simulink model "myCellCharacterizationVerify"  (R2023a)
settings: Solver=daessc  StartTime=0.0  StopTime=2400  MaxStep=1  RelTol=1e-3  AbsTol=1e-3
InitFcn:
  | cellData=load('batt_BatteryCharacterizationResults_3s4p_2RC_20230929_1552.mat');fitData = cellData.battParameters{1,3};cellCapacity = cellData.battParameters{1,2};
undefined symbols (not defined in the file or in its folder): battery_builder_rtmsupport, gcbh
libraries: myPackFromBlock_lib x6, fl_lib x3, nesl_utility x3
CloseFcn:
  | clear fitData
settings Model: Creator=The MathWorks, Inc.  LastModifiedBy=paofu
settings SolverCC: AutoScaleAbsTol=off  AlgebraicLoopSolver=TrustRegion  MinimalZcImpactIntegration=on  MaxZcPerStep=1
settings OptimizationCC: ReuseModelBlockBuffer=off
settings DebuggingCC: ReadBeforeWriteMsg=DisableAll  WriteAfterWriteMsg=DisableAll  WriteAfterReadMsg=DisableAll  MultiTaskDSMMsg=none  UnconnectedInputMsg=warning  UnconnectedOutputMsg=warning  UnconnectedLineMsg=warning  SymbolicDimsDataTypeCodeGenerationDiagnostic=none
settings ModelReferenceCC: UpdateModelReferenceTargets=IfOutOfDate  EnableRefExpFcnMdlSchedulingChecks=on
settings SFSimCC: SFSimEcho=off  CustomCodeUndefinedFunction=UseInterfaceOnly
settings RTWCC: DLArmComputeVersion=19.05
settings SimscapeCC: SimscapeLogType=all  SimscapeLogSimulationStatistics=on  SimscapeLogName=simlog_CellCharacterizationVerify  SimscapeLogDataHistory=10000

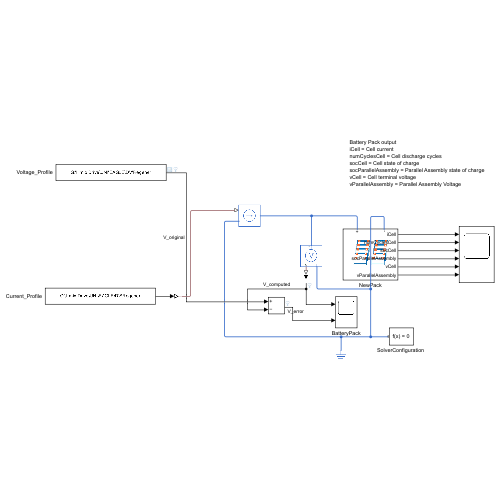
[thumbnail: Simulink's stored preview of the top-level diagram]
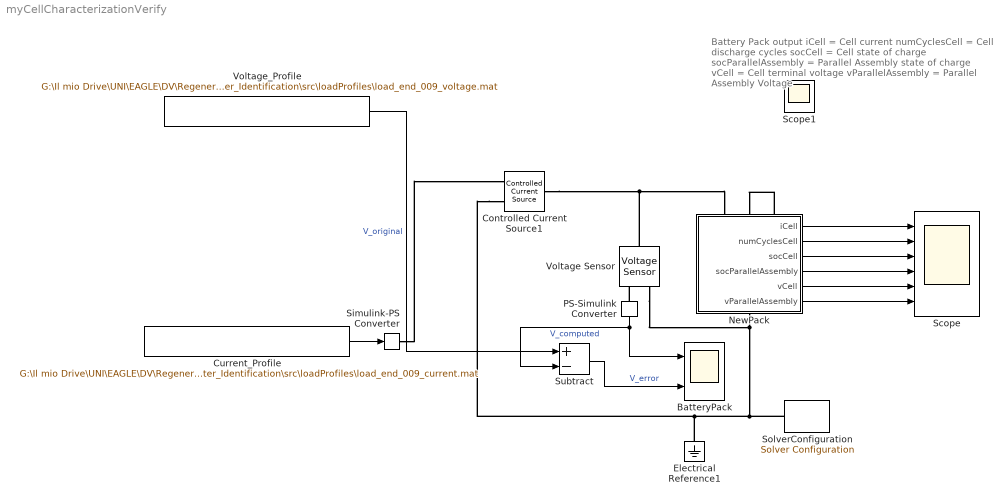
== system myCellCharacterizationVerify ==
  note: Battery Pack output
      | iCell = Cell current
      | numCyclesCell = Cell discharge cycles
      | socCell = Cell state of charge
      | socParallelAssembly = Parallel Assembly state of charge
      | vCell = Cell terminal voltage
      | vParallelAssembly = Parallel Assembly Voltage
  BatteryPack : Scope  NumInputPorts=2
  Controlled Current Source1 : fl_lib/Electrical/Electrical Sources/Controlled Current Source
  Current_Profile : FromFile  FileName=G:\Il mio Drive\UNI\EAGLE\DV\Regenerative-Braking-Development\MATLAB\Parameter_Identification\src\loadProfiles\load_end_009_current.mat  SampleTime=0
  Electrical Reference1 : fl_lib/Electrical/Electrical Elements/Electrical Reference
  NewPack : Subsystem  LoadFcn=battery_builder_rtmsupport('loadfcn',gcbh);
      settings: CopyFcn=battery_builder_rtmsupport('copyfcn',gcbh);  PreCopyFcn=battery_builder_rtmsupport('precopyfcn',gcbh);  PreDeleteFcn=battery_builder_rtmsupport('predeletefcn',gcbh);  PortSchema="{\"entries\":[{\"content\":{\"sides\":[{\"content\":{\"connectorIds\":[\"LConn1\",\"LConn2\"]},\"type\":\"ConnectorPlacement.EquallySpacedRectSide\",\"uuid\":\"66086b7d-23cd-42c5-ba93-ecc496197d21\"},{\"content\":{\"side\":\"RIGHT\"},\"type\":\"ConnectorPlacement.EquallySpacedRectSide\",\"uuid\":\"5adac210-02d4-41ca-984c-4f933a9ee7b3\"},{\"content\":{\"side\":\"TOP\"},\"type\":\"ConnectorPlacement.EquallySpacedRectSide\",\"uuid\":\"5928a5bb-4e09-460c-90ed-8eef0369e6eb\"},{\"content\":{\"connectorIds\":[\"Out1\",\"Out2\",\"Out3\",\"Out4\",\"Out5\",\"Out6\"],\"side\":\"BOTTOM\"},\"type\":\"ConnectorPlacement.EquallySpacedRectSide\",\"uuid\":\"b51498ad-47de-436d-ad23-9534549e135d\"}]},\"type\":\"ConnectorPlacement.EquallySpacedConnector\",\"uuid\":\"4448a3cb-869d-481a-9f4f-41a9fd16508a\"}],\"packageUris\":[\"http://schema.mathworks.com/mf0/Connector/R2020b\"],\"version\":\"1.0\"}"
      mask Display: image('$imagefile')
  PS-Simulink Converter : nesl_utility/PS-Simulink Converter  PhysicalDomain=network_engine_domain  SubClassName=ps_output  LeftPortType=input  RightPortType=output  PseudoPeriodic=off  Frequencies=[]  VectorFormat=inherit  Unit=inherit  AffineConversion=off
  Scope : Scope  NumInputPorts=6
  Simulink-PS Converter : nesl_utility/Simulink-PS Converter  PhysicalDomain=network_engine_domain  SubClassName=ps_input  LeftPortType=input  RightPortType=output  PseudoPeriodic=off  Frequencies=[]  NoiseDistribution=none  NoiseParameters=[]  Unit=1  AffineConversion=off  FilteringAndDerivatives=provide  SimscapeFilterOrder=1  InputFilterTimeConstant=0.001  UdotUserProvided=0
  "SolverConfiguration " : nesl_utility/Solver Configuration  PhysicalDomain=network_engine_domain  SubClassName=solver  LeftPortType=input  RightPortType=generic  Tones=[]  Harmonics=[]  SimulateNoise=off  Profile=off  UseLocalSampling=off  EnableSwitchedLinearOptims=on  FrequencyDomain=off  UseCCode=off  RelTol=0.001  AbsTol=1e-06  MinStep=1e-09  ToWorkspace=off  RevertToSquareIcSolve=off  NumHomotopyIterations=100  PhasorMode=off  PhasorModeNumHarmonics=1  ConsistencySolver=NEWTON_XTOL_AFTER_FTOL  IndexReductionMethod=DerivativeReplacement  DoDC=off  ResidualTolerance=1e-09  ConsistencyTolSource=GLOBAL  ConsistencyAbsTol=0.001  ConsistencyRelTol=0.001  ConsistencyTolFactor=0.001  UseLocalSolver=off  LocalSolverChoice=NE_BACKWARD_EULER_ADVANCER  ResolveIndetEquations=on  FunctionEvalNumThread=1  LocalSolverSampleTime=0.001  DoFixedCost=off  MaxNonlinIter=3  MaxModeIter=2  ComputeImpulses=off  ImpulseIterations=2  LinearAlgebra=auto  LinearAlgebraNumThread=0  EquationFormulation=NE_TIME_EF  DelaysMemoryBudget=1024  AutomaticFiltering=on  FilteringTimeConstant=0.001  PartitionStorageMethod=AS_NEEDED  PartitionMemoryBudget=1024  PartitionMethod=ROBUST
  Subtract : Sum  Inputs=+-
  Voltage Sensor : fl_lib/Electrical/Electrical Sensors/Voltage Sensor
  Voltage_Profile : FromFile  FileName=G:\Il mio Drive\UNI\EAGLE\DV\Regenerative-Braking-Development\MATLAB\Parameter_Identification\src\loadProfiles\load_end_009_voltage.mat  SampleTime=0
  Scope1 : Scope
  wires:
  NewPack/1(iCell) -> Scope/1
  NewPack/2(numCyclesCell) -> Scope/2
  NewPack/3(socCell) -> Scope/3
  NewPack/4(socParallelAssembly) -> Scope/4
  NewPack/5(vCell) -> Scope/5
  NewPack/6(vParallelAssembly) -> Scope/6
  Current_Profile/1 -> Simulink-PS Converter/1
  PS-Simulink Converter/1 -> BatteryPack/1, Subtract/2  "V_computed"
  Subtract/1 -> BatteryPack/2  "V_error"
  Voltage_Profile/1 -> Subtract/1  "V_original"
  connections:
  Controlled Current Source1/RConn2 -- Electrical Reference1/LConn1 -- Voltage Sensor/RConn2 -- NewPack/LConn2 -- "SolverConfiguration "/RConn1
  Simulink-PS Converter/RConn1 -- Controlled Current Source1/RConn1
  Voltage Sensor/LConn1 -- Controlled Current Source1/LConn1 -- NewPack/LConn1
  PS-Simulink Converter/LConn1 -- Voltage Sensor/RConn1

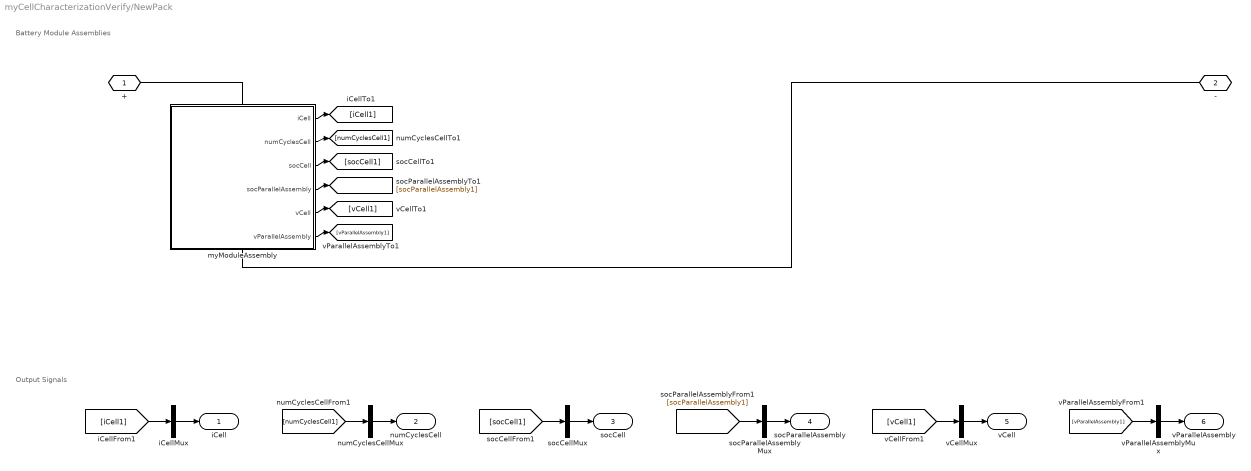
== system myCellCharacterizationVerify/NewPack ==
  note: Battery Module Assemblies
  note: Output Signals
  iCellMux : Mux  Inputs=1
  myModuleAssembly : Subsystem  LoadFcn=battery_builder_rtmsupport('loadfcn',gcbh);
      settings: CopyFcn=battery_builder_rtmsupport('copyfcn',gcbh);  PreCopyFcn=battery_builder_rtmsupport('precopyfcn',gcbh);  PreDeleteFcn=battery_builder_rtmsupport('predeletefcn',gcbh);  PortSchema="{\"entries\":[{\"content\":{\"sides\":[{\"content\":{\"connectorIds\":[\"LConn1\"]},\"type\":\"ConnectorPlacement.EquallySpacedRectSide\",\"uuid\":\"66086b7d-23cd-42c5-ba93-ecc496197d21\"},{\"content\":{\"connectorIds\":[\"RConn1\"],\"side\":\"RIGHT\"},\"type\":\"ConnectorPlacement.EquallySpacedRectSide\",\"uuid\":\"5adac210-02d4-41ca-984c-4f933a9ee7b3\"},{\"content\":{\"side\":\"TOP\"},\"type\":\"ConnectorPlacement.EquallySpacedRectSide\",\"uuid\":\"5928a5bb-4e09-460c-90ed-8eef0369e6eb\"},{\"content\":{\"connectorIds\":[\"Out1\",\"Out2\",\"Out3\",\"Out4\",\"Out5\",\"Out6\"],\"side\":\"BOTTOM\"},\"type\":\"ConnectorPlacement.EquallySpacedRectSide\",\"uuid\":\"b19a6cd0-397b-400c-bc99-badf0012d139\"}]},\"type\":\"ConnectorPlacement.EquallySpacedConnector\",\"uuid\":\"4448a3cb-869d-481a-9f4f-41a9fd16508a\"}],\"packageUris\":[\"http://schema.mathworks.com/mf0/Connector/R2020b\"],\"version\":\"1.0\"}"
      mask Display: image('$imagefile')
  numCyclesCellMux : Mux  Inputs=1
  socCellMux : Mux  Inputs=1
  socParallelAssemblyMux : Mux  Inputs=1
  vCellMux : Mux  Inputs=1
  vParallelAssemblyMux : Mux  Inputs=1
  + : PMIOPort  Side=Left
  - : PMIOPort  Port=2  Side=Left
  iCell : Outport
  numCyclesCell : Outport  Port=2
  socCell : Outport  Port=3
  socParallelAssembly : Outport  Port=4
  vCell : Outport  Port=5
  vParallelAssembly : Outport  Port=6
  wires:
  myModuleAssembly/1(iCell) -> [iCell1]
  iCellMux/1 -> iCell/1
  [iCell1] -> iCellMux/1
  myModuleAssembly/2(numCyclesCell) -> [numCyclesCell1]
  numCyclesCellMux/1 -> numCyclesCell/1
  [numCyclesCell1] -> numCyclesCellMux/1
  myModuleAssembly/3(socCell) -> [socCell1]
  socCellMux/1 -> socCell/1
  [socCell1] -> socCellMux/1
  myModuleAssembly/4(socParallelAssembly) -> [socParallelAssembly1]
  socParallelAssemblyMux/1 -> socParallelAssembly/1
  [socParallelAssembly1] -> socParallelAssemblyMux/1
  myModuleAssembly/5(vCell) -> [vCell1]
  vCellMux/1 -> vCell/1
  [vCell1] -> vCellMux/1
  myModuleAssembly/6(vParallelAssembly) -> [vParallelAssembly1]
  vParallelAssemblyMux/1 -> vParallelAssembly/1
  [vParallelAssembly1] -> vParallelAssemblyMux/1
  connections:
  myModuleAssembly/LConn1 -- +/RConn1
  myModuleAssembly/RConn1 -- -/RConn1

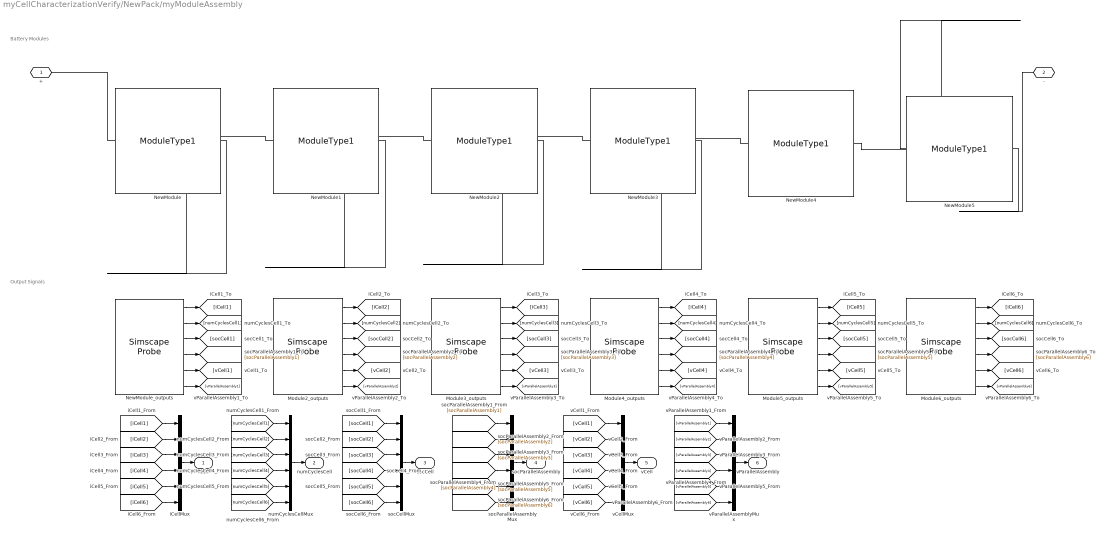
== system myCellCharacterizationVerify/NewPack/myModuleAssembly ==
  note: Output Signals
  note: Battery Modules
  Module2_outputs : SimscapeProbe  BoundBlock=328  Variables={iCell, numCyclesCell, socCell, socParallelAssembly, vCell, vParallelAssembly}
  Module3_outputs : SimscapeProbe  BoundBlock=329  Variables={iCell, numCyclesCell, socCell, socParallelAssembly, vCell, vParallelAssembly}
  Module4_outputs : SimscapeProbe  BoundBlock=330  Variables={iCell, numCyclesCell, socCell, socParallelAssembly, vCell, vParallelAssembly}
  Module5_outputs : SimscapeProbe  BoundBlock=331  Variables={iCell, numCyclesCell, socCell, socParallelAssembly, vCell, vParallelAssembly}
  Module6_outputs : SimscapeProbe  BoundBlock=332  Variables={iCell, numCyclesCell, socCell, socParallelAssembly, vCell, vParallelAssembly}
  NewModule{,1..5} (6 alike) : myPackFromBlock_lib/Modules/ModuleType1  SOC_vecCell=fitData.SOC  V0_vecCell=fitData.V0 V  V_rangeCell=[0, inf] V  R0_vecCell=(fitData.R0_charge + fitData.R0_discharge)/2 Ohm  AHCell=cellCapacity A*hr  extrapolation_optionCell=simscape.enum.extrapolation.nearest  R1_vecCell=fitData.R1 Ohm  tau1_vecCell=fitData.Tau1 s  R2_vecCell=fitData.R2 Ohm  tau2_vecCell=fitData.Tau2 s  P=1  S=6  iCell_specify=off  iCell_priority=None  iCell=0 A  iCell_nominal_specify=off  iCell_nominal_unit=A  iCell_nominal_value=1  vCell_specify=off  vCell_priority=None  vCell=0 V  vCell_nominal_specify=off  vCell_nominal_unit=V  vCell_nominal_value=1  socCell_specify=off  socCell_priority=High  socCell=1  socCell_nominal_specify=off  socCell_nominal_unit=1  socCell_nominal_value=1  numCyclesCell_specify=off  numCyclesCell_priority=High  numCyclesCell=0  numCyclesCell_nominal_specify=off  numCyclesCell_nominal_unit=1  numCyclesCell_nominal_value=1  vParallelAssembly_specify=off  vParallelAssembly_priority=None  vParallelAssembly=repmat(0, 6, 1) V  vParallelAssembly_nominal_specify=off  vParallelAssembly_nominal_unit=V  vParallelAssembly_nominal_value=1  socParallelAssembly_specify=off  socParallelAssembly_priority=None  socParallelAssembly=repmat(1, 6, 1)  socParallelAssembly_nominal_specify=off  socParallelAssembly_nominal_unit=1  socParallelAssembly_nominal_value=1
      settings: InternalSimscapePortConfiguration="{\"Bottom\":[{\"id\":\"n\",\"label\":\"-\",\"type\":\"foundation.electrical.electrical\"}],\"Left\":[],\"Right\":[],\"Top\":[{\"id\":\"p\",\"label\":\"+\",\"type\":\"foundation.electrical.electrical\"}]}"
  NewModule_outputs : SimscapeProbe  BoundBlock=213  Variables={iCell, numCyclesCell, socCell, socParallelAssembly, vCell, vParallelAssembly}
  iCellMux : Mux  Inputs=6
  numCyclesCellMux : Mux  Inputs=6
  socCellMux : Mux  Inputs=6
  socParallelAssemblyMux : Mux  Inputs=6
  vCellMux : Mux  Inputs=6
  vParallelAssemblyMux : Mux  Inputs=6
  + : PMIOPort  Side=Left
  - : PMIOPort  Port=2  Side=Right
  iCell : Outport
  numCyclesCell : Outport  Port=2
  socCell : Outport  Port=3
  socParallelAssembly : Outport  Port=4
  vCell : Outport  Port=5
  vParallelAssembly : Outport  Port=6
  wires:
  [vParallelAssembly6] -> vParallelAssemblyMux/6
  Module6_outputs/6 -> [vParallelAssembly6]
  [vCell6] -> vCellMux/6
  Module6_outputs/5 -> [vCell6]
  [socParallelAssembly6] -> socParallelAssemblyMux/6
  Module6_outputs/4 -> [socParallelAssembly6]
  [socCell6] -> socCellMux/6
  Module6_outputs/3 -> [socCell6]
  [numCyclesCell6] -> numCyclesCellMux/6
  Module6_outputs/2 -> [numCyclesCell6]
  [iCell6] -> iCellMux/6
  Module6_outputs/1 -> [iCell6]
  [vParallelAssembly5] -> vParallelAssemblyMux/5
  [vCell5] -> vCellMux/5
  [socParallelAssembly5] -> socParallelAssemblyMux/5
  [socCell5] -> socCellMux/5
  [numCyclesCell5] -> numCyclesCellMux/5
  [iCell5] -> iCellMux/5
  [vParallelAssembly4] -> vParallelAssemblyMux/4
  [vCell4] -> vCellMux/4
  [socParallelAssembly4] -> socParallelAssemblyMux/4
  [socCell4] -> socCellMux/4
  [numCyclesCell4] -> numCyclesCellMux/4
  [iCell4] -> iCellMux/4
  [vParallelAssembly3] -> vParallelAssemblyMux/3
  [vCell3] -> vCellMux/3
  [socParallelAssembly3] -> socParallelAssemblyMux/3
  [socCell3] -> socCellMux/3
  [numCyclesCell3] -> numCyclesCellMux/3
  [iCell3] -> iCellMux/3
  [vParallelAssembly2] -> vParallelAssemblyMux/2
  [vCell2] -> vCellMux/2
  [socParallelAssembly2] -> socParallelAssemblyMux/2
  [socCell2] -> socCellMux/2
  [numCyclesCell2] -> numCyclesCellMux/2
  [iCell2] -> iCellMux/2
  [vParallelAssembly1] -> vParallelAssemblyMux/1
  vParallelAssemblyMux/1 -> vParallelAssembly/1
  NewModule_outputs/6 -> [vParallelAssembly1]
  [vCell1] -> vCellMux/1
  vCellMux/1 -> vCell/1
  NewModule_outputs/5 -> [vCell1]
  [socParallelAssembly1] -> socParallelAssemblyMux/1
  socParallelAssemblyMux/1 -> socParallelAssembly/1
  NewModule_outputs/4 -> [socParallelAssembly1]
  [socCell1] -> socCellMux/1
  socCellMux/1 -> socCell/1
  NewModule_outputs/3 -> [socCell1]
  [numCyclesCell1] -> numCyclesCellMux/1
  numCyclesCellMux/1 -> numCyclesCell/1
  NewModule_outputs/2 -> [numCyclesCell1]
  [iCell1] -> iCellMux/1
  iCellMux/1 -> iCell/1
  NewModule_outputs/1 -> [iCell1]
  Module2_outputs/1 -> [iCell2]
  Module2_outputs/2 -> [numCyclesCell2]
  Module2_outputs/3 -> [socCell2]
  Module2_outputs/4 -> [socParallelAssembly2]
  Module2_outputs/5 -> [vCell2]
  Module2_outputs/6 -> [vParallelAssembly2]
  Module3_outputs/1 -> [iCell3]
  Module3_outputs/2 -> [numCyclesCell3]
  Module3_outputs/3 -> [socCell3]
  Module3_outputs/4 -> [socParallelAssembly3]
  Module3_outputs/5 -> [vCell3]
  Module3_outputs/6 -> [vParallelAssembly3]
  Module4_outputs/1 -> [iCell4]
  Module4_outputs/2 -> [numCyclesCell4]
  Module4_outputs/3 -> [socCell4]
  Module4_outputs/4 -> [socParallelAssembly4]
  Module4_outputs/5 -> [vCell4]
  Module4_outputs/6 -> [vParallelAssembly4]
  Module5_outputs/1 -> [iCell5]
  Module5_outputs/2 -> [numCyclesCell5]
  Module5_outputs/3 -> [socCell5]
  Module5_outputs/4 -> [socParallelAssembly5]
  Module5_outputs/5 -> [vCell5]
  Module5_outputs/6 -> [vParallelAssembly5]
  connections:
  -/RConn1 -- NewModule5/RConn1
  NewModule/LConn1 -- +/RConn1
  NewModule4/RConn1 -- NewModule5/LConn1
  NewModule4/LConn1 -- NewModule3/RConn1
  NewModule3/LConn1 -- NewModule2/RConn1
  NewModule2/LConn1 -- NewModule1/RConn1
  NewModule1/LConn1 -- NewModule/RConn1
